simulink model "simulacao_com_regulador"  (R2020a)
settings: Solver=ode45  StartTime=0.0  StopTime=5.0  RelTol=1e-3  EnableMultiTasking=on
values from neighbouring files (symbols this model uses):
  C = [1 0]    [trabalho_final.m]
  delta = mb*L*L + Ib    (= 0.00848237644)    [trabalho_final.m]
  g = 9.81    [trabalho_final.m]
  gamah = mb*L    (= 0.039903)    [trabalho_final.m]
  K = place(phi, gama, polos)    [trabalho_final.m]
  Kec = inv(phi)*Kep    [trabalho_final.m]
  Ta = 2*pi/ws    [trabalho_final.m]
undefined symbols (not defined in the file or in its folder): gama, phi
settings Model: Creator=arthu  LastModifiedBy=Acer
settings DataIOCC: LimitDataPoints=on  SaveFormat=Array  ReturnWorkspaceOutputs=off
settings OptimizationCC: LifeSpan=inf
settings DebuggingCC: SFUnexpectedBacktrackingDiag=warning  SFNoUnconditionalDefaultTransitionDiag=warning  SFExecutionAtInitializationDiag=none  ArithmeticOperatorsInVariantConditions=warning
settings HardwareCC: ProdBitPerPointer=32  ProdBitPerSizeT=32  ProdBitPerPtrDiffT=32  ProdLargestAtomicFloat=None  ProdIntDivRoundTo=Undefined  ProdEndianess=Unspecified  ProdWordSize=32  ProdHWDeviceType=32-bit Generic
settings ModelReferenceCC: PropagateSignalLabelsOutOfModel=off
settings SFSimCC: SimUseLocalCustomCode=off  CustomCodeUndefinedFunction=UseInterfaceOnly
settings RTWCC: RTWUseLocalCustomCode=off
settings CodeAppCC: StateflowObjectComments=on
settings GRTTargetCC: TargetLangStandard=C89/C90 (ANSI)
settings ConfigComp: CovMetricSettings=dw  CovHtmlReporting=on  CovSaveCumulativeToWorkspaceVar=on  CovSaveSingleToWorkspaceVar=on  CovExternalEMLEnable=off

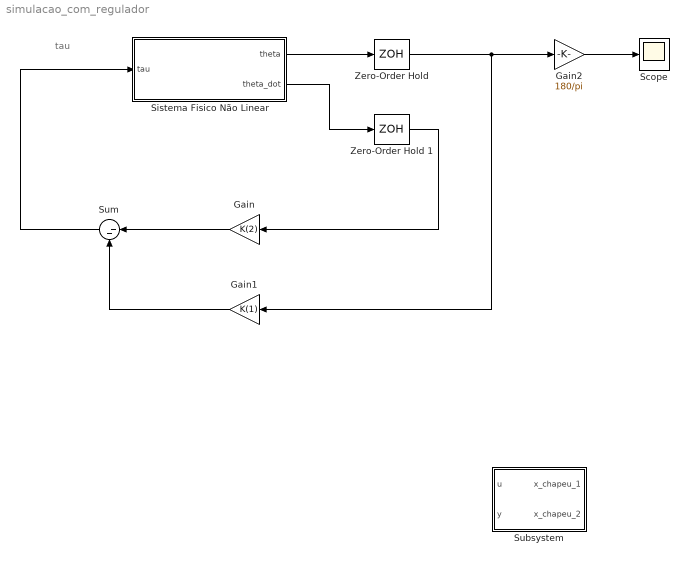
== system simulacao_com_regulador ==
  note: tau
  Gain : Gain  Gain=K(2)
  Gain1 : Gain  Gain=K(1)
  Gain2 : Gain  Gain=180/pi
  "Scope " : Scope
  Sistema Fisico Não Linear : Subsystem
  Subsystem : Subsystem
  Sum : Sum  Inputs=|--
  Zero-Order Hold : ZeroOrderHold  SampleTime=Ta
  Zero-Order Hold 1 : ZeroOrderHold  SampleTime=Ta
  wires:
  Sistema Fisico Não Linear/1(theta) -> Zero-Order Hold/1
  Sistema Fisico Não Linear/2(theta_dot) -> Zero-Order Hold 1/1
  Zero-Order Hold 1/1 -> Gain/1
  Zero-Order Hold/1 -> Gain2/1, Gain1/1
  Gain/1 -> Sum/1
  Gain1/1 -> Sum/2
  Sum/1 -> Sistema Fisico Não Linear/1(tau)
  Gain2/1 -> "Scope "/1

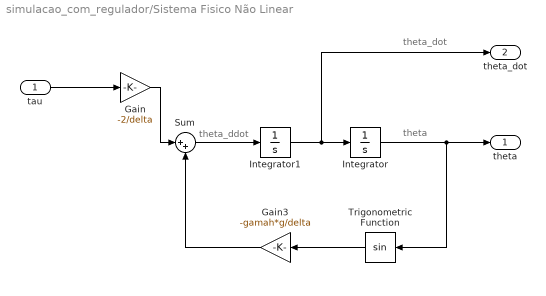
== system simulacao_com_regulador/Sistema Fisico Não Linear ==
  note: theta
  note: theta_dot
  note: theta_ddot
  tau : Inport
  Gain : Gain  Gain=-2/delta
  Gain3 : Gain  Gain=-gamah*g/delta
  Integrator : Integrator  InitialCondition=1
  Integrator1 : Integrator
  Sum : Sum  Inputs=|++
  Trigonometric Function : Trigonometry
  theta : Outport
  theta_dot : Outport  Port=2
  wires:
  tau/1 -> Gain/1
  Sum/1 -> Integrator1/1
  Gain3/1 -> Sum/2
  Integrator/1 -> theta/1, Trigonometric Function/1
  Trigonometric Function/1 -> Gain3/1
  Gain/1 -> Sum/1
  Integrator1/1 -> theta_dot/1, Integrator/1

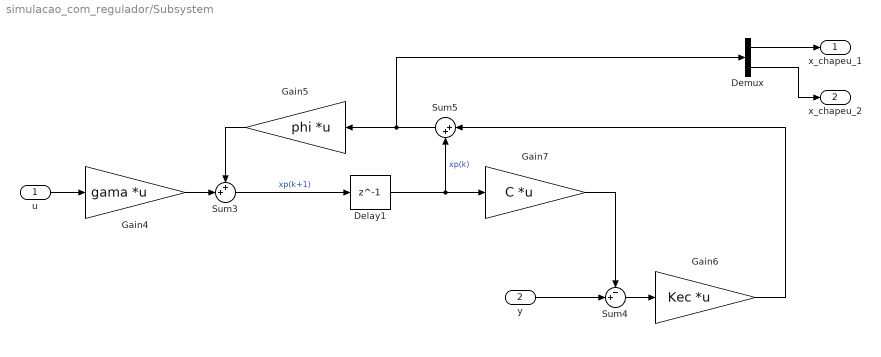
== system simulacao_com_regulador/Subsystem ==
  u : Inport
  y : Inport  Port=2
  Delay1 : Delay  DelayLength=1  InitialCondition=[0;0]
  Demux : Demux  Outputs=2
  Gain4 : Gain  Gain=gama  Multiplication=Matrix(K*u) (u vector)
  Gain5 : Gain  Gain=phi  Multiplication=Matrix(K*u) (u vector)
  Gain6 : Gain  Gain=Kec  Multiplication=Matrix(K*u) (u vector)
  Gain7 : Gain  Gain=C  Multiplication=Matrix(K*u) (u vector)
  Sum3 : Sum  Inputs=++|
  Sum4 : Sum  Inputs=-+|
  Sum5 : Sum  Inputs=|++
  x_chapeu_1 : Outport  VectorParamsAs1DForOutWhenUnconnected=off
  x_chapeu_2 : Outport  Port=2  VectorParamsAs1DForOutWhenUnconnected=off
  wires:
  Gain6/1 -> Sum5/1
  Sum3/1 -> Delay1/1  "xp(k+1)"
  u/1 -> Gain4/1
  Sum5/1 -> Demux/1, Gain5/1
  Gain4/1 -> Sum3/2
  Delay1/1 -> Gain7/1, Sum5/2  "xp(k)"
  Gain5/1 -> Sum3/1
  Sum4/1 -> Gain6/1
  Gain7/1 -> Sum4/1
  y/1 -> Sum4/2
  Demux/1 -> x_chapeu_1/1
  Demux/2 -> x_chapeu_2/1
